simulink model "Symmetry_Inverter_imagined"  (Simulink 8.1)
settings: Solver=ode23t  StartTime=0.0  StopTime=tfin  RelTol=1e-4
values from neighbouring files (symbols this model uses):
  amp_feedback_saturation = 400    [Symmetry_ini_COPY.m]
  Butterworth_filter_order = 8    [Symmetry_ini_COPY.m]
  initial_value = [0.00,0.00,0.00,                  0,0,0]    [Symmetry_ini_COPY.m]
  k_symmetrcal_gain = 1e1    (= 10)    [Symmetry_ini_COPY.m]
  L_Network = [3.185e-3, 3.185e-3, 3.185e-3, 3.185e-3]    [Symmetry_ini_COPY.m]
  L_Source = [3.185e-3, 3.185e-3, 3.185e-3]    [Symmetry_ini_COPY.m]
  Load_R = [50,50,50]    [Symmetry_ini_COPY.m]
  Load_RL = [35.35,   35.35,   35.35;                   0.1125,  0.1125,  0.1125]    [Symmetry_ini_COPY.m]
  NetworkBreaker = [1e5,1e5,1e5,1e5]    [Symmetry_ini_COPY.m]
  P_gain = 5e-5    (= 5e-05)    [Symmetry_ini_COPY.m]
  phase_feedback_saturation = pi    (= 3.14159265359)    [Symmetry_ini_COPY.m]
  Phase_Source = [0,-2/3*pi,-4/3*pi]    [Symmetry_ini_COPY.m]
  PowerGain = [1e-5,1e-5,0]    [Symmetry_ini_COPY.m]
  PV_Power_Capacity = 5e3    (= 5000)    [Symmetry_ini_COPY.m]
  R_Source = [0.4, 0.4, 0.4]    [Symmetry_ini_COPY.m]
  sample = 10e-5    (= 0.0001)    [Symmetry_ini_COPY.m]    (also in animated_norms.m)
  Source_Frequency = [50,50,50]    [Symmetry_ini_COPY.m]
  Start_Control = 0.5    [Symmetry_ini_COPY.m]
  step_size = [1,1,1,                  0.08,0.08,0.08]    [Symmetry_ini_COPY.m]
  test_step = [0.5,0.5,0.5,                  0.02,0.02,0.02]    [Symmetry_ini_COPY.m]
  TransformerBreaker = [1e5,1e5,1e5;                     1e5,1e5,1e5]    [Symmetry_ini_COPY.m]
  Urms_Source = [230,230,230]    [Symmetry_ini_COPY.m]
undefined symbols (not defined in the file or in its folder): Capacitive_Load_RC, START_Load, Wire_resistence
libraries: powerlib x55, simulink x18, dspsigops x10, commsequence2 x6, powerlib_extras x6, dspxfrm3 x3, dsparch4 x3
(part 2 of 2)

== system Symmetry_Inverter_imagined/Synchroniser_Inverter/Current Control/controller/amp_control_T ==
  Control : Inport
  k : Inport  Port=2
  Cp3 : simulink/Logic and Bit Operations/Compare To Constant  relop===  const=5  OutDataTypeStr=uint8  ZeroCross=off
  Delay : UnitDelay  SampleTime=0.001
  Delay4 : UnitDelay  SampleTime=0.02
  Demux2 : Demux  Outputs=5
  I Controller : dspsigops/Sample and Hold  trig=Rising edge  initCond=0  latchinput=off
  I3 Step : Constant  Value=step_size(3)
  "I3 init " : Constant  Value=initial_value(3)
  I3 test step : Constant  Value=test_step(3)
  Mask : simulink/Sources/Repeating Sequence Stair  OutValues=[0 0 1 0 0 0].'  tsamp=mask_sample  OutMin=[]  OutMax=[]  OutDataTypeStr=float('double')  OutputDataTypeScalingMode=Specify via dialog  OutDataType=float('double')  ConRadixGroup=Best Precision: Vector-wise  OutScaling=2^-12
  Product : Product  RndMeth=Zero
  Product12 : Product  RndMeth=Zero
  Product4 : Product  Inputs=4  RndMeth=Zero
  Product8 : Product  Inputs=5  RndMeth=Zero
  Saturation : Saturate  UpperLimit=amp_feedback_saturation  LowerLimit=-amp_feedback_saturation
  Sum : Sum  Inputs=|++
  Sum5 : Sum  Inputs=+++
  amp_T : Outport
  wires:
  Control/1 -> Demux2/1
  Product12/1 -> amp_T/1
  Product8/1 -> Sum/1
  Delay/1 -> Saturation/1
  "I3 init "/1 -> Sum5/2
  Delay4/1 -> Sum5/3
  Demux2/5 -> Product8/2
  Demux2/4 -> Product/2
  Demux2/3 -> Product4/3, Product8/1
  Demux2/2 -> Product4/2
  Demux2/1 -> Product12/1, Product8/4
  I3 Step/1 -> Product8/3
  Cp3/1 -> I Controller/Trigger
  Mask/1 -> Product/1, Product4/4
  Sum5/1 -> Product12/2
  I3 test step/1 -> Product4/1
  I Controller/1 -> Delay4/1, Delay/1
  Product4/1 -> Sum5/1
  Product/1 -> Cp3/1
  Sum/1 -> I Controller/1
  Saturation/1 -> Sum/2
  k/1 -> Product8/5

== system Symmetry_Inverter_imagined/Synchroniser_Inverter/Current Control/controller/phase_control_R ==
  Control : Inport
  Cp3 : simulink/Logic and Bit Operations/Compare To Constant  relop===  const=5  OutDataTypeStr=uint8  ZeroCross=off
  Delay : UnitDelay  SampleTime=0.001
  Delay4 : UnitDelay  SampleTime=0.02
  Demux2 : Demux  Outputs=5
  I Controller : dspsigops/Sample and Hold  trig=Rising edge  initCond=0  latchinput=off
  I3 Step : Constant  Value=step_size(4)
  "I3 init " : Constant  Value=initial_value(4)
  I3 test step : Constant  Value=test_step(4)
  Mask : simulink/Sources/Repeating Sequence Stair  OutValues=[0 0 0 1 0 0].'  tsamp=mask_sample  OutMin=[]  OutMax=[]  OutDataTypeStr=float('double')  OutputDataTypeScalingMode=Specify via dialog  OutDataType=float('double')  ConRadixGroup=Best Precision: Vector-wise  OutScaling=2^-12
  Product : Product  RndMeth=Zero
  Product12 : Product  RndMeth=Zero
  Product4 : Product  Inputs=4  RndMeth=Zero
  Product8 : Product  Inputs=4  RndMeth=Zero
  Saturation : Saturate  UpperLimit=phase_feedback_saturation  LowerLimit=-phase_feedback_saturation
  Sum : Sum  Inputs=|++
  Sum5 : Sum  Inputs=+++
  phase_R : Outport
  wires:
  Saturation/1 -> Sum/2
  Sum/1 -> I Controller/1
  Product/1 -> Cp3/1
  Product4/1 -> Sum5/1
  I Controller/1 -> Delay/1, Delay4/1
  I3 test step/1 -> Product4/1
  Sum5/1 -> Product12/2
  Mask/1 -> Product4/4, Product/1
  Cp3/1 -> I Controller/Trigger
  I3 Step/1 -> Product8/3
  Demux2/1 -> Product12/1, Product8/4
  Demux2/2 -> Product4/2
  Demux2/3 -> Product8/1, Product4/3
  Demux2/4 -> Product/2
  Demux2/5 -> Product8/2
  Delay4/1 -> Sum5/3
  "I3 init "/1 -> Sum5/2
  Delay/1 -> Saturation/1
  Product8/1 -> Sum/1
  Product12/1 -> phase_R/1
  Control/1 -> Demux2/1

== system Symmetry_Inverter_imagined/Synchroniser_Inverter/Current Control/controller/phase_control_T ==
  Control : Inport
  Cp3 : simulink/Logic and Bit Operations/Compare To Constant  relop===  const=5  OutDataTypeStr=uint8  ZeroCross=off
  Delay : UnitDelay  SampleTime=0.001
  Delay4 : UnitDelay  SampleTime=0.02
  Demux2 : Demux  Outputs=5
  I Controller : dspsigops/Sample and Hold  trig=Rising edge  initCond=0  latchinput=off
  I3 Step : Constant  Value=step_size(6)
  "I3 init " : Constant  Value=initial_value(6)
  I3 test step : Constant  Value=test_step(6)
  Mask : simulink/Sources/Repeating Sequence Stair  OutValues=[0 0 0 0 0 1].'  tsamp=mask_sample  OutMin=[]  OutMax=[]  OutDataTypeStr=float('double')  OutputDataTypeScalingMode=Specify via dialog  OutDataType=float('double')  ConRadixGroup=Best Precision: Vector-wise  OutScaling=2^-12
  Product : Product  RndMeth=Zero
  Product12 : Product  RndMeth=Zero
  Product4 : Product  Inputs=4  RndMeth=Zero
  Product8 : Product  Inputs=4  RndMeth=Zero
  Saturation : Saturate  UpperLimit=phase_feedback_saturation  LowerLimit=-phase_feedback_saturation
  Sum : Sum  Inputs=|++
  Sum5 : Sum  Inputs=+++
  phase_S : Outport
  wires:
  Saturation/1 -> Sum/2
  Sum/1 -> I Controller/1
  Product/1 -> Cp3/1
  Product4/1 -> Sum5/1
  I Controller/1 -> Delay/1, Delay4/1
  I3 test step/1 -> Product4/1
  Sum5/1 -> Product12/2
  Mask/1 -> Product4/4, Product/1
  Cp3/1 -> I Controller/Trigger
  I3 Step/1 -> Product8/3
  Demux2/1 -> Product12/1, Product8/4
  Demux2/2 -> Product4/2
  Demux2/3 -> Product8/1, Product4/3
  Demux2/4 -> Product/2
  Demux2/5 -> Product8/2
  Delay4/1 -> Sum5/3
  "I3 init "/1 -> Sum5/2
  Delay/1 -> Saturation/1
  Product8/1 -> Sum/1
  Product12/1 -> phase_S/1
  Control/1 -> Demux2/1

== system Symmetry_Inverter_imagined/Synchroniser_Inverter/Current Control/Current_Sources/Conncection_Measurements/3_Phase_P_Q ==
  U_abc : Inport
  I_abc : Inport  Port=2
  Demux1 : Demux  Outputs=3
  Demux3 : Demux  Outputs=3
  P Q in3 : powerlib_extras/Measurements/Active & Reactive Power  f1=Source_Frequency(1)
  P Q in4 : powerlib_extras/Measurements/Active & Reactive Power  f1=Source_Frequency(2)
  P Q in5 : powerlib_extras/Measurements/Active & Reactive Power  f1=Source_Frequency(3)
  PQ_R : Outport
  PQ_S : Outport  Port=2
  PQ_T : Outport  Port=3
  wires:
  P Q in3/1 -> PQ_R/1
  P Q in4/1 -> PQ_S/1
  P Q in5/1 -> PQ_T/1
  Demux3/1 -> P Q in3/1
  Demux3/2 -> P Q in4/1
  Demux3/3 -> P Q in5/1
  Demux1/1 -> P Q in3/2
  Demux1/2 -> P Q in4/2
  Demux1/3 -> P Q in5/2
  U_abc/1 -> Demux3/1
  I_abc/1 -> Demux1/1

== matlab function Synchroniser_Inverter/Calculate_Norms/Mearusement_calc/geometrial norm ==
  data: amplitude_R input double; GEO_norm output double; amplitude_S input double; amplitude_T input double; phase_R input double; phase_S input double; phase_T input double
function GEO_norm = fcn(amplitude_R,amplitude_S,amplitude_T,phase_R,phase_S,phase_T)
%#codegen

x1=[0,0,0,0];
y1=[0,0,0,0];
x2=[0,0,0,0];
y2=[0,0,0,0];

GEO_norm=0;

coder.extrinsic('geometry_solver')

        %% Ideal parameters
        Amplitude_1=[325.3,325.3,325.3];                     %[V]
        %Phase_1=[-1.5855,2.6033,0.5089];
        Phase_1=[0,-2/3*pi,-4/3*pi];                     %[rad]
      
        %% Real parameters
        Amplitude_2=[amplitude_R,amplitude_S,amplitude_T];
        Phase_2=[phase_R,phase_S,phase_T];
        %Extension of the vectors with the first element to get closed triangles on
        %plots and for use as polygons
        Amplitude_1_ex=[Amplitude_1 Amplitude_1(1)];
        Phase_1_ex=[Phase_1 Phase_1(1)];
        Amplitude_2_ex=[Amplitude_2 Amplitude_2(1)];
        Phase_2_ex=[Phase_2 Phase_2(1)];
        
        GEO_norm=geometry_solver(Amplitude_1_ex, Phase_1_ex, Amplitude_2_ex, Phase_2_ex);

== matlab function Synchroniser_Inverter/Calculate_Norms/Mearusement_calc/vectorial norm old ==
  data: amplitude_R input double; VEC_norm output double; amplitude_S input double; amplitude_T input double; phase_R input double; phase_S input double; phase_T input double
function VEC_norm = fcn(amplitude_R,amplitude_S,amplitude_T,phase_R,phase_S,phase_T)
%#codegen

  
   N=complex(0);
   V_real=complex([0,0,0]');
  %V_012=complex([0,0,0]');
   V_real(1)=amplitude_R.*exp(1i*phase_R);
   V_real(2)=amplitude_S.*exp(1i*phase_S);
   V_real(3)=amplitude_T.*exp(1i*phase_T); 

   R_error=230*exp(1j*-0/360*2*pi)  -V_real(1);
   S_error=230*exp(1j*-120/360*2*pi)-V_real(2);
   T_error=230*exp(1j*-240/360*2*pi)-V_real(3);
   %VEC_norm=abs(R_error*S_error)+abs(R_error*T_error)+abs(S_error*T_error);
   N=R_error*S_error+R_error*T_error+S_error*T_error;
   VEC_norm=abs(N);

== matlab function Synchroniser_Inverter/Calculate_Norms/Mearusement_calc/regular norm ==
  data: amplitude_R input double; REG_norm output double; amplitude_S input double; amplitude_T input double; phase_R input double; phase_S input double; phase_T input double
function REG_norm = fcn(amplitude_R,amplitude_S,amplitude_T,phase_R,phase_S,phase_T)
%#codegen

 A=(1/3)*[1,                1,                  1;...
          1,      exp(1i*120/360*2*pi),        exp(1i*240/360*2*pi);...
          1,      exp(1i*240/360*2*pi),       exp(1i*120/360*2*pi)];
   
   V_real=complex([0,0,0]');
   V_012=complex([0,0,0]');
   V_real(1)=amplitude_R.*exp(1i*phase_R);
   V_real(2)=amplitude_S.*exp(1i*phase_S);
   V_real(3)=amplitude_T.*exp(1i*phase_T); 
   V_012=A*V_real;
   REG_norm=(abs(V_012(3))/abs(V_012(2)))*100;

== matlab function Synchroniser_Inverter/Current Control/controller/MATLAB Function1 ==
  data: amp input double; CC output double; phase input double; t input double
function CC = fcn(amp,phase,t)
%#codegen

CC = zeros(3,1);
CC_mtx=[amp(1),50,phase(1),0;...
        amp(1),50,phase(1)-2/3*pi,0;...
        amp(1),50,phase(1)-4/3*pi,0];
% T=1;
% CC=[(CC_mtx(1,1)*sin(2*pi*CC_mtx(1,2)*t+CC_mtx(1,3))+CC_mtx(1,4)).*(1-exp(-t/T)),...
%     (CC_mtx(2,1)*sin(2*pi*CC_mtx(2,2)*t+CC_mtx(2,3))+CC_mtx(2,4)).*(1-exp(-t/T)),...
%     (CC_mtx(3,1)*sin(2*pi*CC_mtx(3,2)*t+CC_mtx(3,3))+CC_mtx(3,4)).*(1-exp(-t/T))]';

CC=[(CC_mtx(1,1)*sin(2*pi*CC_mtx(1,2)*t+CC_mtx(1,3))+CC_mtx(1,4)),...
    (CC_mtx(2,1)*sin(2*pi*CC_mtx(2,2)*t+CC_mtx(2,3))+CC_mtx(2,4)),...
    (CC_mtx(3,1)*sin(2*pi*CC_mtx(3,2)*t+CC_mtx(3,3))+CC_mtx(3,4))]';

== matlab function Synchroniser_Inverter/Current Control/controller/MATLAB Function ==
  data: amp input double; CC output double; phase input double; t input double
function CC = fcn(amp,phase,t)
%#codegen
CC = zeros(3,1);

CC_mtx=[amp(1),50,phase(1),0;...
        amp(2),50,phase(2),0;...
        amp(3),50,phase(3),0];
% T=1;
% CC=[(CC_mtx(1,1)*sin(2*pi*CC_mtx(1,2)*t+CC_mtx(1,3))+CC_mtx(1,4)).*(1-exp(-t/T)),...
%     (CC_mtx(2,1)*sin(2*pi*CC_mtx(2,2)*t+CC_mtx(2,3))+CC_mtx(2,4)).*(1-exp(-t/T)),...
%     (CC_mtx(3,1)*sin(2*pi*CC_mtx(3,2)*t+CC_mtx(3,3))+CC_mtx(3,4)).*(1-exp(-t/T))]';

CC=[(CC_mtx(1,1)*sin(2*pi*CC_mtx(1,2)*t+CC_mtx(1,3))+CC_mtx(1,4)),...
    (CC_mtx(2,1)*sin(2*pi*CC_mtx(2,2)*t+CC_mtx(2,3))+CC_mtx(2,4)),...
    (CC_mtx(3,1)*sin(2*pi*CC_mtx(3,2)*t+CC_mtx(3,3))+CC_mtx(3,4))]';

== matlab function Synchroniser_Inverter/Calculate_Norms/Mearusement_calc/geometrial norm meaned ==
  data: amplitude_R input double; GEO_norm output double; amplitude_S input double; amplitude_T input double; phase_R input double; phase_S input double; phase_T input double; Mean output double
function [GEO_norm,Mean] = fcn(amplitude_R,amplitude_S,amplitude_T,phase_R,phase_S,phase_T)
%#codegen

x1=[0,0,0,0];
y1=[0,0,0,0];
x2=[0,0,0,0];
y2=[0,0,0,0];

GEO_norm=0;
Mean=0;

coder.extrinsic('geometry_solver')

        %% Ideal parameters
        Mean=(amplitude_R+amplitude_S+amplitude_T)/3;
        Amplitude_1=[Mean,Mean,Mean];                     %[V]
        %Phase_1=[-1.5855,2.6033,0.5089];
        Phase_1=[0,-2/3*pi,-4/3*pi];                     %[rad]
      
        %% Real parameters
        Amplitude_2=[amplitude_R,amplitude_S,amplitude_T];
        Phase_2=[phase_R,phase_S,phase_T];
        %Extension of the vectors with the first element to get closed triangles on
        %plots and for use as polygons
        Amplitude_1_ex=[Amplitude_1 Amplitude_1(1)];
        Phase_1_ex=[Phase_1 Phase_1(1)];
        Amplitude_2_ex=[Amplitude_2 Amplitude_2(1)];
        Phase_2_ex=[Phase_2 Phase_2(1)];
        
        GEO_norm=geometry_solver(Amplitude_1_ex, Phase_1_ex, Amplitude_2_ex, Phase_2_ex);

== matlab function Synchroniser_Inverter/Calculate_Norms/Mearusement_calc/vectorial norm new ==
  data: amplitude_R input double; VEC_norm output double; amplitude_S input double; amplitude_T input double; phase_R input double; phase_S input double; phase_T input double
function VEC_norm = fcn(amplitude_R,amplitude_S,amplitude_T,phase_R,phase_S,phase_T)
%#codegen

  
   N=complex(0);
   V_real=complex([0,0,0]');
  %V_012=complex([0,0,0]');
   V_real(1)=amplitude_R.*exp(1i*phase_R);
   V_real(2)=amplitude_S.*exp(1i*phase_S);
   V_real(3)=amplitude_T.*exp(1i*phase_T); 

   R_error=230*exp(1j*-0/360*2*pi)  -V_real(1);
   S_error=230*exp(1j*-120/360*2*pi)-V_real(2);
   T_error=230*exp(1j*-240/360*2*pi)-V_real(3);
   VEC_norm=abs(R_error*S_error)+abs(R_error*T_error)+abs(S_error*T_error);
   %N=R_error*S_error+R_error*T_error+S_error*T_error;
   %VEC_norm=abs(N);

== matlab function Synchroniser_Inverter/Calculate_Norms/Mearusement_calc/vectorial norm old meaned ==
  data: amplitude_R input double; VEC_norm output double; amplitude_S input double; amplitude_T input double; phase_R input double; phase_S input double; phase_T input double; Mean output double
function [VEC_norm,Mean] = fcn(amplitude_R,amplitude_S,amplitude_T,phase_R,phase_S,phase_T)
%#codegen

   Mean=0;
   Mean=(amplitude_R+amplitude_S+amplitude_T)/3;
   N=complex(0);
   V_real=complex([0,0,0]');
  %V_012=complex([0,0,0]');
   V_real(1)=Mean.*exp(1i*phase_R);
   V_real(2)=Mean.*exp(1i*phase_S);
   V_real(3)=Mean.*exp(1i*phase_T); 

   R_error=230*exp(1j*-0/360*2*pi)  -V_real(1);
   S_error=230*exp(1j*-120/360*2*pi)-V_real(2);
   T_error=230*exp(1j*-240/360*2*pi)-V_real(3);
   %VEC_norm=abs(R_error*S_error)+abs(R_error*T_error)+abs(S_error*T_error);
   N=R_error*S_error+R_error*T_error+S_error*T_error;
   VEC_norm=abs(N);

== matlab function Synchroniser_Inverter/Calculate_Norms/Mearusement_calc/vectorial norm new meaned ==
  data: amplitude_R input double; VEC_norm output double; amplitude_S input double; amplitude_T input double; phase_R input double; phase_S input double; phase_T input double; Mean output double
function [VEC_norm,Mean] = fcn(amplitude_R,amplitude_S,amplitude_T,phase_R,phase_S,phase_T)
%#codegen

  
   Mean=0;
   Mean=(amplitude_R+amplitude_S+amplitude_T)/3;
   N=complex(0);
   V_real=complex([0,0,0]');
  %V_012=complex([0,0,0]');
   V_real(1)=Mean.*exp(1i*phase_R);
   V_real(2)=Mean.*exp(1i*phase_S);
   V_real(3)=Mean.*exp(1i*phase_T);  

   R_error=230*exp(1j*-0/360*2*pi)  -V_real(1);
   S_error=230*exp(1j*-120/360*2*pi)-V_real(2);
   T_error=230*exp(1j*-240/360*2*pi)-V_real(3);
   VEC_norm=abs(R_error*S_error)+abs(R_error*T_error)+abs(S_error*T_error);
   %N=R_error*S_error+R_error*T_error+S_error*T_error;
   %VEC_norm=abs(N);
